simulink model "decouple_state_lqr"  (R2022a)
settings: Solver=VariableStepAuto  StartTime=0.0  StopTime=50  RelTol=1e-3
values from neighbouring files (symbols this model uses):
  A = [0 0 0 1 0 0 ... (first row only)    [main.m]
  B = [0 0 ... (first row only)    [main.m]
  C2 = [1 0 0 0 0 0 ... (first row only)    [main.m]
  F = inv(Bx)    [main.m]
  kdecoup = F*Cxx    [main.m]
  klqr2 = real(inv(R)*B'*P2)    [main.m]
settings Model: Creator=wyton  LastModifiedBy=dzsgy
settings SolverCC: AlgebraicLoopSolver=TrustRegion
settings DebuggingCC: UnconnectedInputMsg=warning  UnconnectedOutputMsg=warning  UnconnectedLineMsg=warning  SFMachineParentedDataDiag=warning

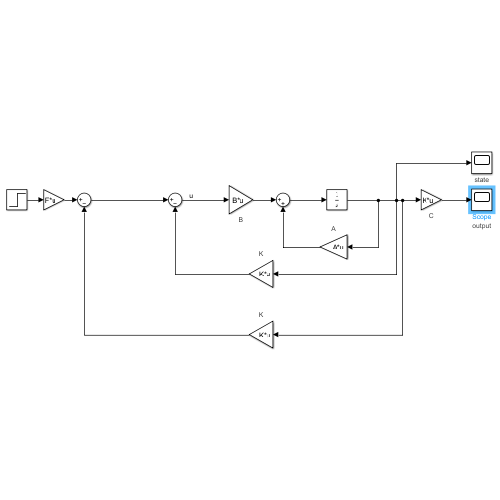
[thumbnail: Simulink's stored preview of the top-level diagram]
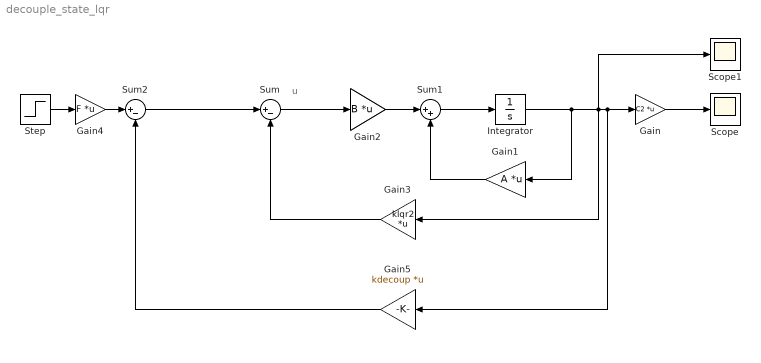
== system decouple_state_lqr ==
  note: u
  Gain : Gain  Gain=C2  Multiplication=Matrix(K*u)
      settings: AttributesFormatString=C
  Gain1 : Gain  Gain=A  Multiplication=Matrix(K*u)
      settings: AttributesFormatString=A
  Gain2 : Gain  Tag=B  Gain=B  Multiplication=Matrix(K*u)
      settings: AttributesFormatString=B
  Gain3 : Gain  Gain=klqr2  Multiplication=Matrix(K*u)
      settings: AttributesFormatString=K
  Gain4 : Gain  Gain=F  Multiplication=Matrix(K*u)
  Gain5 : Gain  Gain=kdecoup  Multiplication=Matrix(K*u)
      settings: AttributesFormatString=K
  Integrator : Integrator
  Scope : Scope
      settings: AttributesFormatString=output
  Scope1 : Scope
      settings: AttributesFormatString=state
  Step : Step  Time=0  After=[1,0]  SampleTime=0
  Sum : Sum  Inputs=|+-
  Sum1 : Sum  Inputs=|++
  Sum2 : Sum  Inputs=|+-
  wires:
  Sum/1 -> Gain2/1
  Sum1/1 -> Integrator/1
  Gain2/1 -> Sum1/1
  Integrator/1 -> Gain1/1, Gain3/1, Gain5/1, Gain/1, Scope1/1
  Gain1/1 -> Sum1/2
  Gain/1 -> Scope/1
  Gain3/1 -> Sum/2
  Gain5/1 -> Sum2/2
  Sum2/1 -> Sum/1
  Step/1 -> Gain4/1
  Gain4/1 -> Sum2/1
